simulink model "EngBrk_Tst"  (R2016b)
settings: configuration reference "CodeGenConfigSet" (kept outside this file)
settings Model: Creator=lenovo  LastModifiedBy=lenovo
settings ConfigSetRef: SourceLocation=Base Workspace

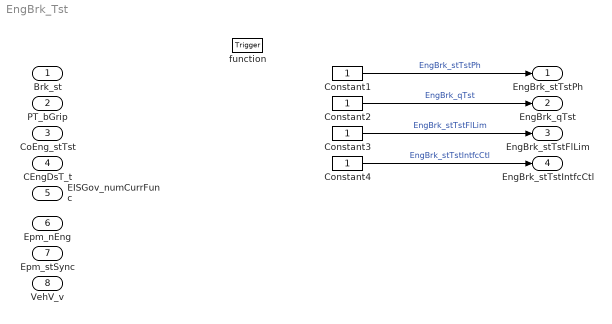
== system EngBrk_Tst ==
  Brk_st : Inport  Description=Brake switch state  OutMin=0  OutMax=255  OutDataTypeStr=State
  PT_bGrip : Inport  Description=Grip is for sure present (the converter lockup clutch / the automated or manual clutch is completely closed and PT_bNoGrip = FALSE)  Port=2  OutMin=0  OutMax=1  OutDataTypeStr=boolean
  CoEng_stTst : Inport  Description=Engine test state  Port=3  OutMin=0  OutMax=255  OutDataTypeStr=State
  CEngDsT_t : Inport  Tag=deg  Description=Coolant temperature  Port=4  OutMin=-50  OutMax=200  OutDataTypeStr=Temp_deg
  EISGov_numCurrFunc : Inport  Description=|  Port=5  OutDataTypeStr=Enum: EISGov_num_conv
      | Identification name / number of the currently active
      | EISGov client, which determines the current
      | controller parameters
  Epm_nEng : Inport  Tag=rpm  Description=Engine speed  Port=6  OutMin=0  OutMax=6000  OutDataTypeStr=EngSpeed_rpm
  Epm_stSync : Inport  Description=State of synchronization  Port=7  OutDataTypeStr=Enum: EpmSynState_conv
  VehV_v : Inport  Tag=km/h  Description=Vehicle speed  Port=8  OutMin=0  OutMax=255  OutDataTypeStr=VehSpeed_km_h
  function : TriggerPort  TriggerType=function-call  VariantControl=Variant
  Constant1 : Constant  OutDataTypeStr=State
  Constant2 : Constant  OutDataTypeStr=FuelMass_mg_hub
  Constant3 : Constant  OutDataTypeStr=State
  Constant4 : Constant  OutDataTypeStr=State
  EngBrk_stTstPh : Outport  Description=State of the engine brake test state machine  OutMin=0  OutMax=255  OutDataTypeStr=State
  EngBrk_qTst : Outport  Tag=mg/hub  Description=Fuel quantity to be used during the engine brake test mghub  Port=2  OutMin=-319  OutMax=319  OutDataTypeStr=FuelMass_mg_hub
  EngBrk_stTstFlLim : Outport  Description=Status for the limitation of the engine brake test fuel quantity by the fuel quantity out of CoEng_trqInrCurrLim  Port=3  OutMin=0  OutMax=255  OutDataTypeStr=State
  EngBrk_stTstIntfcCtl : Outport  Description=Status of engine brake test interface with peripheral modules  Port=4  OutMin=0  OutMax=255  OutDataTypeStr=State
  wires:
  Constant1/1 -> EngBrk_stTstPh/1  "EngBrk_stTstPh"
  Constant2/1 -> EngBrk_qTst/1  "EngBrk_qTst"
  Constant3/1 -> EngBrk_stTstFlLim/1  "EngBrk_stTstFlLim"
  Constant4/1 -> EngBrk_stTstIntfcCtl/1  "EngBrk_stTstIntfcCtl"
